simulink model "simulation_ff"  (R2018b)
settings: Solver=VariableStepAuto  StartTime=0.0  StopTime=10.0  RelTol=1e-5  AbsTol=1e-9
libraries: cstblocks x2
settings Model: Creator=daniel  LastModifiedBy=daniel

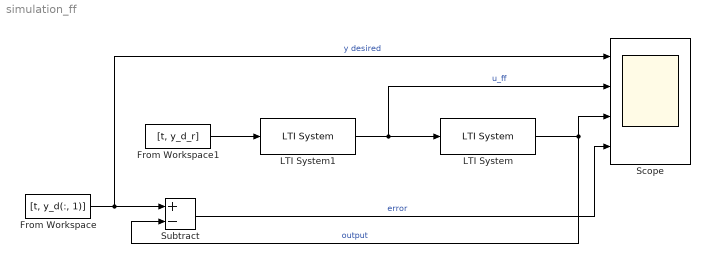
== system simulation_ff ==
  From Workspace : FromWorkspace  VariableName=[t, y_d(:, 1)]  SampleTime=0
  From Workspace1 : FromWorkspace  VariableName=[t, y_d_r]  SampleTime=0
  LTI System : cstblocks/LTI System  sys=sys_err  IC=[]
  LTI System1 : cstblocks/LTI System  sys=sys_inv  IC=0
  Scope : Scope  NumInputPorts=4
  Subtract : Sum  Inputs=+-
  wires:
  From Workspace/1 -> Scope/1, Subtract/1  "y desired"
  From Workspace1/1 -> LTI System1/1
  Subtract/1 -> Scope/4  "error"
  LTI System/1 -> Scope/3, Subtract/2  "output"
  LTI System1/1 -> LTI System/1, Scope/2  "u_ff"
